simulink model "Terje2"  (Simulink 7.5)
settings: Solver=VariableStepDiscrete  StartTime=0.0  StopTime=10.0  RelTol=1e-3
settings Model: Creator=Terje B  LastModifiedBy=Terje B
settings DebuggingCC: StrictBusMsg=Warning

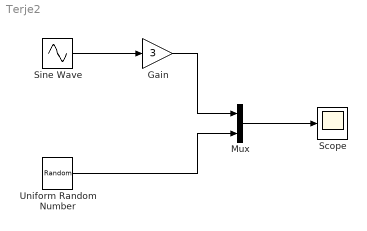
== system Terje2 ==
  Gain : Gain  Gain=3  ParameterDataType=fixdt(1, 16)  ParameterScaling=2^0  OutDataType=fixdt(1, 16)  OutScaling=2^0
  Mux : Mux  Inputs=2
  Scope : Scope
  Sine Wave : Sin  Amplitude=1  Bias=0  Frequency=5  Phase=0  Samples=10  SampleTime=0  Offset=0
  Uniform Random Number : UniformRandomNumber  SampleTime=0.1
  wires:
  Sine Wave/1 -> Gain/1
  Gain/1 -> Mux/1
  Uniform Random Number/1 -> Mux/2
  Mux/1 -> Scope/1
